simulink library "LinkLib"  (R2023b)
settings: Solver=VariableStepAuto  StartTime=0.0  StopTime=10.0  RelTol=1e-3
undefined symbols (not defined in the file): LpinL, X, Y, Z
libraries: sm_lib x73, $bdroot x2
(part 1 of 3)
settings Model: Creator=abirdas  LastModifiedBy=abirdas

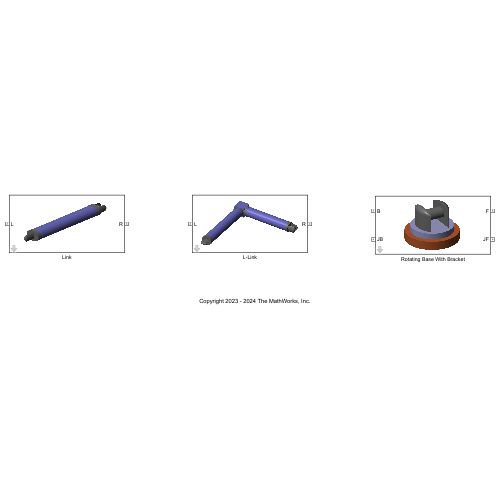
[thumbnail: Simulink's stored preview of the top-level diagram]
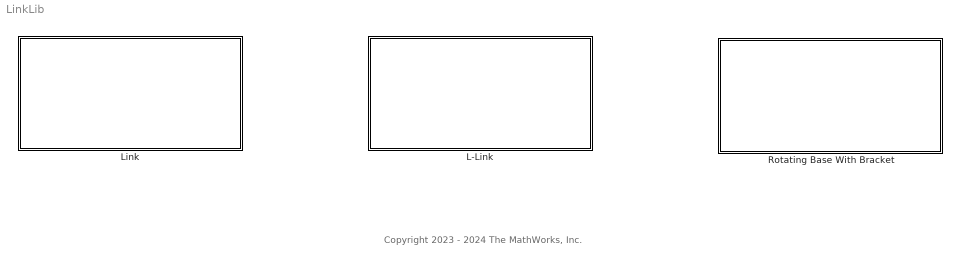
== system LinkLib ==
  note: Copyright 2023 - 2024 The MathWorks, Inc.
  L-Link : Subsystem  mask(Robot Arm L-Link){connConfigLLLink=Single bracket, oriLLLink=+X, connConfigRLLink=Double bracket with pin, oriRLLink=+Z, linkRadius=0.01, member1TotalLength=0.1, member2TotalLength=0.2, inertiaType=Custom, linkMass=0.1, linkCM=[0 0 0], linkMOI=[1 1 1], linkPOI=[0 0 0], linkDensity=7780, linkColor=[0.5 0.5 0.9]}
      mask prompts: connConfigLLLink "Left connector configuration"; oriLLLink "Left bracket orientation"; connConfigRLLink "Right connector configuration"; oriRLLink "Right bracket orientation"; linkRadius "Link radius (m)"; member1TotalLength "Member1 total length (m)"; member2TotalLength "Member 2 total length (m)"; inertiaType "Inertia type"; linkMass "Mass (kg)"; linkCM "Center of mass (m)"; linkMOI "Moments of inertia (kg*m^2)"; linkPOI "Products of inertia (kg*m^2)"; linkDensity "Link density (kg/m^3)"; linkColor "Link color"
      mask help:
      | Consists of two perpendicular members rigidly connected to one another using a rigid middle connector. Each member represents a robot arm link that consists of a middle section, two end plates (left plate and right plate) and two end connectors (left connector and right connector). These components are rigidly connected to one another. The first member or Member 1 is a link with No connector as the right connector. The second member or Member 2 is a link with No connector as the left connector.
      |
      | Attachment points are:
      | L: Left connector
      | R: Right connector
      |
      | Connectors can be of following types:
      | No connector
      | Single bracket
      | Double bracket with pin
      | Rotating pin
      | Pin socket
      |
      | Where
      | Link radius: Radius of the cylinders that constitute the middle section of the links representing Member 1 and Member 2
      | Member1 total length: Distance between the center of left connector of Member 1 and the center of rigid middle connector
      | Member2 total length: Distance between the center of rigid middle connector and the center of right connector of Member 2
      mask init:
      | linkRadius = get_param(gcb,'value@linkRadius');
      | member1TotalLength = get_param(gcb,'value@member1TotalLength');
      | member1Path = [gcb,'/Member 1'];
      | member2TotalLength = get_param(gcb,'value@member2TotalLength');
      | member2Path = [gcb,'/Member 2'];
      | rigidMiddleConnPath = [gcb,'/Rigid Middle Connector'];
      | member1Length = member1TotalLength - 1.05*linkRadius;
      | middleConnL = 2*1.05*linkRadius;
      | set_param(member1Path,'linkRadius',num2str(linkRadius));
      | set_param(member1Path,'linkLength',num2str(member1Length));
      | set_param(rigidMiddleConnPath,'midConnL',num2str(middleConnL));
      | member2Length = member2TotalLength - 1.05*linkRadius;
      | set_param(member2Path,'linkRadius',num2str(linkRadius));
      | set_param(member2Path,'linkLength',num2str(member2Length))
      mask Help: web('LLink.html')
      mask TypeOptions connConfigLLLink: No connector | Single bracket | Double bracket with pin | Rotating pin | Pin socket
      mask Callback connConfigLLLink:
      | maskObj = Simulink.Mask.get(gcb);
      | connConfigLLLink = maskObj.getParameter('connConfigLLLink');
      | oriLLLink = maskObj.getParameter('oriLLLink');
      | member1Path = [gcb,'/Member 1'];
      | if strcmp(connConfigLLLink.Value,'No connector') || ...
      |         strcmp(connConfigLLLink.Value,'Rotating pin') || ...
      |         strcmp(connConfigLLLink.Value,'Pin socket')
      |     oriLLLink.Visible = 'off';
      | else
      |     oriLLLink.Visible = 'on';
      | end
      | set_param(member1Path,'connConfigL',connConfigLLLink.Value);
      | set_param(member1Path,'oriL',oriLLLink.Value);
      | set_param(member1Path,'connConfigR','No connector');
      mask TypeOptions oriLLLink: +X | +Z
      mask TypeOptions connConfigRLLink: No connector | Single bracket | Double bracket with pin | Rotating pin | Pin socket
      mask Callback connConfigRLLink:
      | maskObj = Simulink.Mask.get(gcb);
      | connConfigRLLink = maskObj.getParameter('connConfigRLLink');
      | oriRLLink = maskObj.getParameter('oriRLLink');
      | member2Path = [gcb,'/Member 2'];
      | if strcmp(connConfigRLLink.Value,'No connector') || ...
      |         strcmp(connConfigRLLink.Value,'Rotating pin') || ...
      |         strcmp(connConfigRLLink.Value,'Pin socket')
      |     oriRLLink.Visible = 'off';
      | else
      |     oriRLLink.Visible = 'on';
      | end
      | set_param(member2Path,'connConfigR',connConfigRLLink.Value);
      | if strcmp(oriRLLink.Value,'+Z')
      |     set_param(member2Path,'oriR',oriRLLink.Value);
      | elseif strcmp(oriRLLink.Value,'+Y')
      |     set_param(member2Path,'oriR','+X');
      | end
      | set_param(member2Path,'connConfigL','No connector');
      mask TypeOptions oriRLLink: +Y | +Z
      mask TypeOptions inertiaType: Calculate from geometry | Custom
      mask Callback inertiaType:
      | maskObj = Simulink.Mask.get(gcb);
      | inertiaTypeLLink = maskObj.getParameter('inertiaType');
      | massLLink = maskObj.getParameter('linkMass');
      | centerOfMassLLink = maskObj.getParameter('linkCM');
      | momentsOfInertiaLLink = maskObj.getParameter('linkMOI');
      | productsOfInertiaLLink = maskObj.getParameter('linkPOI');
      | linkDensityLLink = maskObj.getParameter('linkDensity');
      | linkColorLLink = maskObj.getParameter('linkColor');
      | linkRadius = maskObj.getParameter('linkRadius');
      | member1Path = [gcb,'/Member 1'];
      | member2Path = [gcb,'/Member 2'];
      | rigidMiddleConnPath = [gcb,'/Rigid Middle Connector/Brick Solid'];
      | if strcmp(inertiaTypeLLink.Value,'Calculate from geometry')
      |     massLLink.Visible='off';
      |     centerOfMassLLink.Visible='off';
      |     momentsOfInertiaLLink.Visible='off';
      |     productsOfInertiaLLink.Visible='off';
      |     linkDensityLLink.Visible='on';
      |     set_param(rigidMiddleConnPath,'InertiaType','CalculateFromGeometry');
      |     set_param(rigidMiddleConnPath,'BasedOnType','Density');
      | elseif strcmp(inertiaTypeLLink.Value,'Custom')
      |     massLLink.Visible='on';
      |     centerOfMassLLink.Visible='on';
      |     momentsOfInertiaLLink.Visible='on';
      |     productsOfInertiaLLink.Visible='on';
      |     linkDensityLLink.Visible='off';
      |     set_param(rigidMiddleConnPath,'InertiaType','Custom');
      | end
      | 
      | set_param(member1Path,'inertiaType',inertiaTypeLLink.Value);
      | set_param(member1Path,'linkMass',massLLink.Value);
      | set_param(member1Path,'linkCM',centerOfMassLLink.Value);
      | set_param(member1Path,'linkMOI',momentsOfInertiaLLink.Value);
      | set_param(member1Path,'linkPOI',productsOfInertiaLLink.Value);
      | set_param(member1Path,'linkDensity',linkDensityLLink.Value);
      | set_param(member1Path,'linkColor',linkColorLLink.Value);
      | set_param(member2Path,'linkRadius',linkRadius.Value);
      | set_param(member2Path,'inertiaType',inertiaTypeLLink.Value);
      | set_param(member2Path,'linkMass','1e-10');
      | set_param(member2Path,'linkCM','[0 0 0]');
      | set_param(member2Path,'linkMOI','[0 0 0]');
      | set_param(member2Path,'linkPOI','[0 0 0]');
      | set_param(member2Path,'linkDensity',linkDensityLLink.Value);
      | set_param(member2Path,'linkColor',linkColorLLink.Value);
      mask DialogControl Container1 Prompt: Connector configuration
      mask DialogControl Container2 Prompt: Geometry
      mask DialogControl Container3 Prompt: Inertia
      mask DialogControl Container4 Prompt: Graphic
      mask Display:
      | image('LLinkIcon.png');
      | port_label('lconn',1,'L');
      | port_label('rconn',1,'R');
  Link : Subsystem  mask(Robot Arm Link){connConfigL=Single bracket, oriL=+X, connConfigR=Double bracket with pin, oriR=+X, linkRadius=0.01, linkLength=0.1, inertiaType=Custom, linkMass=3, linkCM=[0 0 0], linkMOI=[1 1 1], linkPOI=[0 0 0], linkDensity=7780, linkColor=[0.5, 0.5, 0.88]}
      mask prompts: connConfigL "Left connector configuration"; oriL "Left bracket orientation"; connConfigR "Right connector configuration"; oriR "Right bracket orientation"; linkRadius "Link radius (m)"; linkLength "Link length (m)"; inertiaType "Inertia type"; linkMass "Mass (kg)"; linkCM "Center of mass (m)"; linkMOI "Moments of inertia (kg*m^2)"; linkPOI "Products of inertia (kg*m^2)"; linkDensity "Link density (kg//m^3)"; linkColor "Link color"
      mask help:
      | Consists of a cylindrical middle section, two end plates (left plate and right plate) and two end connectors (left connector and right connector). These components are rigidly connected to one another.
      |
      | Attachment points are:
      | L: Left connector
      | R: Right connector
      |
      | Connectors can be of following types:
      | No connector
      | Single bracket
      | Double bracket with pin
      | Rotating pin
      | Pin socket
      |
      | Where
      | Link radius: Radius of the cylinder that constitutes the middle section of the link
      | Link length: Distance between the center of left connector and the center of right connector of the link
      mask init:
      | maskObj = Simulink.Mask.get(gcb);
      | connConfigL = maskObj.getParameter('connConfigL');
      | connConfigR = maskObj.getParameter('connConfigR');
      | linkRadius = get_param(gcb,'value@linkRadius');
      | linkLength = get_param(gcb,'value@linkLength');
      | bracketLength = (linkRadius/2)*1.5;
      | pinLength = linkRadius/2;
      | midSecPath = [gcb,'/Middle Section'];
      | leftPlatePath = [gcb,'/Left Plate'];
      | rightPlatePath = [gcb,'/Right Plate'];
      | if strcmp(connConfigL.Value, 'Single bracket') || strcmp(connConfigL.Value,'Double bracket with pin')
      |     if strcmp(connConfigR.Value, 'Single bracket') || strcmp(connConfigR.Value,'Double bracket with pin')
      |         midSecLength = (linkLength - 2*bracketLength)/(1 + 2*0.05);
      |     elseif strcmp(connConfigR.Value, 'Rotating pin') || strcmp(connConfigR.Value,'Pin socket')
      |         midSecLength= (linkLength - bracketLength - 0.5*pinLength)/(1 + 2*0.05);
      |     elseif strcmp(connConfigR.Value, 'No connector')
      |         midSecLength= (linkLength - bracketLength)/(1 + 2*0.05);
      |     end
      | elseif strcmp(connConfigL.Value, 'Rotating pin') || strcmp(connConfigL.Value,'Pin socket')
      |     if strcmp(connConfigR.Value, 'Single bracket') || strcmp(connConfigR.Value,'Double bracket with pin')
      |         midSecLength= (linkLength - bracketLength - 0.5*pinLength)/(1 + 2*0.05);
      |     elseif strcmp(connConfigR.Value, 'Rotating pin') || strcmp(connConfigR.Value,'Pin socket')
      |         midSecLength = (linkLength - 2*0.5*pinLength)/(1 + 2*0.05);
      |     elseif strcmp(connConfigR.Value, 'No connector')
      |         midSecLength = (linkLength - 0.5*pinLength)/(1 + 2*0.05);
      |     end
      | elseif strcmp(connConfigL.Value, 'No connector')
      |     if strcmp(connConfigR.Value, 'Single bracket') || strcmp(connConfigR.Value,'Double bracket with pin')
      |         midSecLength= (linkLength - bracketLength)/(1 + 2*0.05);
      |     elseif strcmp(connConfigR.Value, 'Rotating pin') || strcmp(connConfigR.Value,'Pin socket')
      |         midSecLength = (linkLength - 0.5*pinLength)/(1 + 2*0.05);
      |     elseif strcmp(connConfigR.Value, 'No connector')
      |         midSecLength = (linkLength)/(1 + 2*0.05);
      |     end
      | end
      | set_param(midSecPath, 'midSecLength', num2str(midSecLength));
      | set_param(leftPlatePath, 'plateThickness', num2str(0.05*midSecLength));
      | set_param(rightPlatePath, 'plateThickness', num2str(0.05*midSecLength));
      mask Help: web('Link.html')
      mask TypeOptions connConfigL: No connector | Single bracket | Double bracket with pin | Rotating pin | Pin socket
      mask Callback connConfigL:
      | maskObj = Simulink.Mask.get(gcb);
      | connConfigL = maskObj.getParameter('connConfigL');
      | oriL = maskObj.getParameter('oriL');
      | blockPath = [gcb,'/Left Connector'];
      | transformBracketPathL = [gcb,'/Left Connector/Bracket/Bracket/Transform Bracket L'];
      | transformBracketPathR = [gcb,'/Left Connector/Bracket/Bracket/Transform Bracket R'];
      | pinBracketPath = [gcb,'/Left Connector/Bracket/Pin B'];
      | if strcmp(connConfigL.Value,'No connector')
      |     oriL.Visible='off';
      |     set_param(blockPath, 'LabelModeActiveChoice', 'NoConnectorL');
      | elseif strcmp(connConfigL.Value,'Single bracket')
      |     oriL.Visible='on';
      |     set_param(blockPath, 'LabelModeActiveChoice', 'BracketL');
      |     set_param(pinBracketPath,'commented','through');
      |     set_param(transformBracketPathL,'TranslationStandardOffset','0');
      |     set_param(transformBracketPathR,'TranslationStandardOffset','0');
      | elseif strcmp(connConfigL.Value,'Double bracket with pin')
      |     oriL.Visible='on';
      |     set_param(blockPath, 'LabelModeActiveChoice', 'BracketL');
      |     set_param(pinBracketPath,'commented','off');
      |     set_param(transformBracketPathL,'TranslationStandardOffset','wBracket/2');
      |     set_param(transformBracketPathR,'TranslationStandardOffset','wBracket/2');
      | elseif strcmp(connConfigL.Value,'Rotating pin')
      |     oriL.Visible='off';
      |     set_param(blockPath, 'LabelModeActiveChoice', 'RotatingPinL');
      | elseif strcmp(connConfigL.Value,'Pin socket')
      |     oriL.Visible='off';
      |     set_param(blockPath, 'LabelModeActiveChoice', 'PinSocketL');
      | end
      mask TypeOptions oriL: +X | +Z
      mask TypeOptions connConfigR: No connector | Single bracket | Double bracket with pin | Rotating pin | Pin socket
      mask Callback connConfigR:
      | maskObj = Simulink.Mask.get(gcb);
      | connConfigR = maskObj.getParameter('connConfigR');
      | oriR = maskObj.getParameter('oriR');
      | blockPath = [gcb,'/Right Connector'];
      | transformBracketPathL = [gcb,'/Right Connector/Bracket/Bracket/Transform Bracket L'];
      | transformBracketPathR = [gcb,'/Right Connector/Bracket/Bracket/Transform Bracket R'];
      | 
      | pinBracketPath = [gcb,'/Right Connector/Bracket/Pin B'];
      | if strcmp(connConfigR.Value,'No connector')
      |     oriR.Visible='off';
      |     set_param(blockPath, 'LabelModeActiveChoice', 'NoConnectorR');
      | elseif strcmp(connConfigR.Value,'Single bracket')
      |     oriR.Visible='on';
      |     set_param(blockPath, 'LabelModeActiveChoice', 'BracketR');
      |     set_param(pinBracketPath,'commented','through');
      |     set_param(transformBracketPathL,'TranslationStandardOffset','0');
      |     set_param(transformBracketPathR,'TranslationStandardOffset','0');
      | elseif strcmp(connConfigR.Value,'Double bracket with pin')
      |     oriR.Visible='on';
      |     set_param(blockPath, 'LabelModeActiveChoice', 'BracketR');
      |     set_param(pinBracketPath,'commented','off');
      |     set_param(transformBracketPathL,'TranslationStandardOffset','wBracket/2');
      |     set_param(transformBracketPathR,'TranslationStandardOffset','wBracket/2');
      | elseif strcmp(connConfigR.Value,'Rotating pin')
      |     oriR.Visible='off';
      |     set_param(blockPath, 'LabelModeActiveChoice', 'RotatingPinR');
      | elseif strcmp(connConfigR.Value,'Pin socket')
      |     oriR.Visible='off';
      |     set_param(blockPath, 'LabelModeActiveChoice', 'PinSocketR');
      | end
      mask TypeOptions oriR: +X | +Z
      mask Callback oriR:
      | maskObj = Simulink.Mask.get(gcb);
      | blockPath = gcb;
      | connConfigL = maskObj.getParameter('connConfigL');
      | connConfigR = maskObj.getParameter('connConfigR');
      | oriR = maskObj.getParameter('oriR');
      | oriL = maskObj.getParameter('oriL');
      | 
      | transformLXPath = [blockPath,'/Transform LX'];
      | transformLZPath = [blockPath,'/Transform LZ'];
      | transformRB1Path = [blockPath,'/Transform RB1'];
      | transformRB2Path = [blockPath,'/Transform RB2'];
      | transformRFPath = [blockPath,'/Transform RF'];
      | 
      | if strcmp(connConfigL.Value,'Single bracket') || ...
      |         strcmp(connConfigL.Value,'Double bracket with pin')
      | if strcmp(connConfigR.Value,'Single bracket') || ...
      |         strcmp(connConfigR.Value,'Double bracket with pin')
      | if strcmp(oriL.Value,'+X') && strcmp(oriR.Value,'+X')
      |     set_param(transformLXPath,'commented','off');
      |     set_param(transformLZPath,'commented','through');
      |     set_param(transformRB1Path,'commented','off');
      |     set_param(transformRB2Path,'commented','through');
      |     set_param(transformRFPath,'commented','off');
      | elseif strcmp(oriL.Value,'+X') && strcmp(oriR.Value,'+Z')
      |     set_param(transformLXPath,'commented','off');
      |     set_param(transformLZPath,'commented','through');
      |     set_param(transformRB1Path,'commented','through');
      |     set_param(transformRB2Path,'commented','off');
      |     set_param(transformRFPath,'commented','through');
      | elseif strcmp(oriL.Value,'+Z') && strcmp(oriR.Value,'+X')
      |     set_param(transformLXPath,'commented','through');
      |     set_param(transformLZPath,'commented','off');
      |     set_param(transformRB1Path,'commented','through');
      |     set_param(transformRB2Path,'commented','off');
      |     set_param(transformRFPath,'commented','off');
      | elseif strcmp(oriL.Value,'+Z') && strcmp(oriR.Value,'+Z')
      |     set_param(transformLXPath,'commented','through');
      |     set_param(transformLZPath,'commented','off');
      |     set_param(transformRB1Path,'commented','off');
      |     set_param(transformRB2Path,'commented','through');
      |     set_param(transformRFPath,'commented','through');
      | end
      | elseif strcmp(connConfigR.Value,'No connector') || ...
      |         strcmp(connConfigR.Value,'Rotating pin') || ...
      |         strcmp(connConfigR.Value,'Pin socket')
      |     if strcmp(oriL.Value,'+X')
      |     set_param(transformLXPath,'commented','off');
      |     set_param(transformLZPath,'commented','through');
      |     set_param(transformRB1Path,'commented','off');
      |     set_param(transformRB2Path,'commented','through');
      |     set_param(transformRFPath,'commented','off');
      |     elseif strcmp(oriL.Value,'+Z')
      |     set_param(transformLXPath,'commented','through');
      |     set_param(transformLZPath,'commented','off');
      |     set_param(transformRB1Path,'commented','through');
      |     set_param(transformRB2Path,'commented','off');
      |     set_param(transformRFPath,'commented','off');
      |     end
      | end
      | elseif strcmp(connConfigL.Value,'No connector') || ...
      |         strcmp(connConfigL.Value,'Rotating pin') || ...
      |         strcmp(connConfigL.Value,'Pin socket')
      |     if strcmp(connConfigR.Value,'Single bracket') || ...
      |         strcmp(connConfigR.Value,'Double bracket with pin')
      |     if strcmp(oriR.Value,'+X')
      |     set_param(transformLXPath,'commented','off');
      |     set_param(transformLZPath,'commented','through');
      |     set_param(transformRB1Path,'commented','off');
      |     set_param(transformRB2Path,'commented','through');
      |     set_param(transformRFPath,'commented','off');
      |     elseif strcmp(oriR.Value,'+Z')
      |     set_param(transformLXPath,'commented','off');
      |     set_param(transformLZPath,'commented','through');
      |     set_param(transformRB1Path,'commented','through');
      |     set_param(transformRB2Path,'commented','off');
      |     set_param(transformRFPath,'commented','through');
      |     end
      | elseif strcmp(connConfigR.Value,'No connector') || ...
      |         strcmp(connConfigR.Value,'Rotating pin') || ...
      |         strcmp(connConfigR.Value,'Pin socket')
      |     set_param(transformLXPath,'commented','off');
      |     set_param(transformLZPath,'commented','through');
      |     set_param(transformRB1Path,'commented','off');
      |     set_param(transformRB2Path,'commented','through');
      |     set_param(transformRFPath,'commented','off');
      |     end
      | end
      mask TypeOptions inertiaType: Calculate from Geometry | Custom
      mask Callback inertiaType:
      | maskObj = Simulink.Mask.get(gcb);
      | inertiaType = maskObj.getParameter('inertiaType');
      | mass = maskObj.getParameter('linkMass');
      | centerOfMass = maskObj.getParameter('linkCM');
      | momentsOfInertia = maskObj.getParameter('linkMOI');
      | productsOfInertia = maskObj.getParameter('linkPOI');
      | linkDensity = maskObj.getParameter('linkDensity');
      | leftBracketLSolid1Path = [gcb,'/Left Connector/Bracket/Bracket/BracketL/Extruded Solid'];
      | leftBracketLSolid2Path = [gcb,'/Left Connector/Bracket/Bracket/BracketL/Revolved Solid'];
      | leftBracketRSolid1Path = [gcb,'/Left Connector/Bracket/Bracket/BracketR/Extruded Solid'];
      | leftBracketRSolid2Path = [gcb,'/Left Connector/Bracket/Bracket/BracketR/Revolved Solid'];
      | leftBracketPinPath = [gcb,'/Left Connector/Bracket/Pin B/Cylindrical Solid'];
      | leftRotatingPinPath = [gcb,'/Left Connector/Rotating Pin/Cylindrical Solid'];
      | leftPinSocketPath = [gcb,'/Left Connector/Pin Socket/Bar'];
      | leftPlatePath = [gcb,'/Left Plate/Cylindrical Solid'];
      | midSecPath = [gcb,'/Middle Section/Cylindrical Solid'];
      | rightPlatePath = [gcb,'/Right Plate/Cylindrical Solid'];
      | rightBracketLSolid1Path = [gcb,'/Right Connector/Bracket/Bracket/BracketL/Extruded Solid'];
      | rightBracketLSolid2Path = [gcb,'/Right Connector/Bracket/Bracket/BracketL/Revolved Solid'];
      | rightBracketRSolid1Path = [gcb,'/Right Connector/Bracket/Bracket/BracketR/Extruded Solid'];
      | rightBracketRSolid2Path = [gcb,'/Right Connector/Bracket/Bracket/BracketR/Revolved Solid'];
      | rightBracketPinPath = [gcb,'/Right Connector/Bracket/Pin B/Cylindrical Solid'];
      | rightRotatingPinPath = [gcb,'/Right Connector/Rotating Pin/Cylindrical Solid'];
      | rightPinSocketPath = [gcb,'/Right Connector/Pin Socket/Bar'];
      | 
      | if strcmp(inertiaType.Value,'Calculate from Geometry')
      |     mass.Visible='off';
      |     centerOfMass.Visible='off';
      |     momentsOfInertia.Visible='off';
      |     productsOfInertia.Visible='off';
      |     linkDensity.Visible='on';
      |     set_param(leftBracketLSolid1Path,'InertiaType','CalculateFromGeometry');
      |     set_param(leftBracketLSolid1Path,'BasedOnType','Density');
      |     set_param(leftBracketLSolid2Path,'InertiaType','CalculateFromGeometry');
      |     set_param(leftBracketLSolid2Path,'BasedOnType','Density');
      |     set_param(leftBracketRSolid1Path,'InertiaType','CalculateFromGeometry');
      |     set_param(leftBracketRSolid1Path,'BasedOnType','Density');
      |     set_param(leftBracketRSolid2Path,'InertiaType','CalculateFromGeometry');
      |     set_param(leftBracketRSolid2Path,'BasedOnType','Density');
      |     set_param(leftBracketPinPath,'InertiaType','CalculateFromGeometry');
      |     set_param(leftBracketPinPath,'BasedOnType','Density');
      |     set_param(leftRotatingPinPath,'InertiaType','CalculateFromGeometry');
      |     set_param(leftRotatingPinPath,'BasedOnType','Density');
      |     set_param(leftPinSocketPath,'InertiaType','CalculateFromGeometry');
      |     set_param(leftPinSocketPath,'BasedOnType','Density');
      |     set_param(leftPlatePath,'InertiaType','CalculateFromGeometry');
      |     set_param(leftPlatePath,'BasedOnType','Density');
      |     set_param(midSecPath,'InertiaType','CalculateFromGeometry');
      |     set_param(midSecPath,'BasedOnType','Density');
      |     set_param(rightPlatePath,'InertiaType','CalculateFromGeometry');
      |     set_param(rightPlatePath,'BasedOnType','Density');
      |     set_param(rightBracketLSolid1Path,'InertiaType','CalculateFromGeometry');
      |     set_param(rightBracketLSolid1Path,'BasedOnType','Density');
      |     set_param(rightBracketLSolid2Path,'InertiaType','CalculateFromGeometry');
      |     set_param(rightBracketLSolid2Path,'BasedOnType','Density');
      |     set_param(rightBracketRSolid1Path,'InertiaType','CalculateFromGeometry');
      |     set_param(rightBracketRSolid1Path,'BasedOnType','Density');
      |     set_param(rightBracketRSolid2Path,'InertiaType','CalculateFromGeometry');
      |     set_param(rightBracketRSolid2Path,'BasedOnType','Density');
      |     set_param(rightBracketPinPath,'InertiaType','CalculateFromGeometry');
      |     set_param(rightBracketPinPath,'BasedOnType','Density');
      |     set_param(rightRotatingPinPath,'InertiaType','CalculateFromGeometry');
      |     set_param(rightRotatingPinPath,'BasedOnType','Density');
      |     set_param(rightPinSocketPath,'InertiaType','CalculateFromGeometry');
      |     set_param(rightPinSocketPath,'BasedOnType','Density');
      | elseif strcmp(inertiaType.Value,'Custom')
      |     mass.Visible='on';
      |     centerOfMass.Visible='on';
      |     momentsOfInertia.Visible='on';
      |     productsOfInertia.Visible='on';
      |     linkDensity.Visible='off';
      |     set_param(leftBracketLSolid1Path,'InertiaType','Custom');
      |     set_param(leftBracketLSolid2Path,'InertiaType','Custom');
      |     set_param(leftBracketRSolid1Path,'InertiaType','Custom');
      |     set_param(leftBracketRSolid2Path,'InertiaType','Custom');
      |     set_param(leftBracketPinPath,'InertiaType','Custom');
      |     set_param(leftRotatingPinPath,'InertiaType','Custom');
      |     set_param(leftPinSocketPath,'InertiaType','Custom');
      |     set_param(leftPlatePath,'InertiaType','Custom');
      |     set_param(midSecPath,'InertiaType','Custom');
      |     set_param(rightPlatePath,'InertiaType','Custom');
      |     set_param(rightBracketLSolid1Path,'InertiaType','Custom');
      |     set_param(rightBracketLSolid2Path,'InertiaType','Custom');
      |     set_param(rightBracketRSolid1Path,'InertiaType','Custom');
      |     set_param(rightBracketRSolid2Path,'InertiaType','Custom');
      |     set_param(rightBracketPinPath,'InertiaType','Custom');
      |     set_param(rightRotatingPinPath,'InertiaType','Custom');
      |     set_param(rightPinSocketPath,'InertiaType','Custom');
      | end
      mask DialogControl Container1 Prompt: Connector configuration
      mask DialogControl Container2 Prompt: Geometry
      mask DialogControl Container3 Prompt: Inertia
      mask DialogControl Container4 Prompt: Graphic
      mask Display:
      | image('LinkIcon.PNG');
      | port_label('lconn',1,'L');
      | port_label('rconn',1,'R');
  Rotating Base With Bracket : Subsystem  mask(Rotating Base With Bracket){connConfig=Single bracket, baseRadius=0.01, baseTotalLength=0.05, baseInertiaType=Custom, baseDensity=7780, baseMass=5, baseCM=[0 0 0], baseMOI=[1 1 1], basePOI=[0 0 0], rotorInertiaType=Custom, rotorDensity=7780, rotorMass=3, rotorCM=[0 0 0], rotorMOI=[1 1 1], rotorPOI=[0 0 0], baseColor=[0.8 0.4 0.2], rotorColor=[0.7 0.7 0.9]}
      mask prompts: connConfig "Bracket configuration"; baseRadius "Fixed base radius (m)"; baseTotalLength "Base total length (m)"; baseInertiaType "Inertia type"; baseDensity "Density (kg/m^3)"; baseMass "Mass (kg)"; baseCM "Center of mass (m)"; baseMOI "Moments of inertia (kg*m^2)"; basePOI "Products of inertia (kg*m^2)"; rotorInertiaType "Inertia type"; rotorDensity "Density (kg/m^3)"; rotorMass "Mass (kg)"; rotorCM "Center of mass (m)"; rotorMOI "Moments of inertia (kg*m^2)"; rotorPOI "Products of inertia (kg*m^2)"; baseColor "Fixed base color"; rotorColor "Rotor color"
      mask help:
      | Consists of a fixed base, a rotor and a bracket mounted on the rotor. The rotor must be connected to the fixed base using a Revolute Joint. The bracket is connected rigidly to the rotor.
      |
      | Attachment points are:
      | B: The bottom of the fixed base
      | F: The center point of the hole or between the two holes of the bracket.
      | JB: The top of the fixed base, which is attached to the bottom of the rotor.
      | JF: The bottom of the rotor, which is attached to the top of the fixed base.
      | All attachments are configured for Revolute joints.
      |
      | Bracket can be of following types:
      | Single bracket
      | Double bracket with pin
      |
      | Where
      | Fixed base radius: Radius of the cylinder that constitutes the fixed base
      | Base total length: Distance between the bottom surface of the fixed base and the center of hole (for Single bracket) or center of pin (for Double bracket with pin) of the bracket, measured in the direction perpendicular to the bottom surface of the fixed base
      mask init:
      | baseTotalLength = get_param(gcb,'value@baseTotalLength');
      | baseRadius = get_param(gcb,'value@baseRadius');
      | rotorRadius = 0.8*baseRadius;
      | bracketLength = (rotorRadius/2)*1.5;
      | baseLength = (baseTotalLength - bracketLength)/1.7;
      | rotorLength = 0.7*baseLength;
      | basePath = [gcb,'/Fixed Base'];
      | rotorPath = [gcb,'/Rotor'];
      | set_param(basePath, 'CylinderLength', num2str(baseLength));
      | set_param(rotorPath, 'CylinderLength', num2str(rotorLength));
      mask Help: web('RotatingBaseWithBracket.html')
      mask TypeOptions connConfig: Double bracket with pin | Single bracket
      mask Callback connConfig:
      | maskObj = Simulink.Mask.get(gcb);
      | connConfig = maskObj.getParameter('connConfig');
      | pinBracketPath = [gcb,'/Bracket/Pin B'];
      | transformBracketPathL = [gcb,'/Bracket/Bracket/Transform Bracket L'];
      | transformBracketPathR = [gcb,'/Bracket/Bracket/Transform Bracket R'];
      | switch connConfig.Value
      |     case 'Single bracket'
      |         set_param(pinBracketPath,'commented','through');
      |         set_param(transformBracketPathL,'TranslationStandardOffset','0');
      |         set_param(transformBracketPathR,'TranslationStandardOffset','0');
      |     case 'Double bracket with pin'
      |         set_param(pinBracketPath,'commented','off');
      |         set_param(transformBracketPathL,'TranslationStandardOffset','wBracket/2');
      |         set_param(transformBracketPathR,'TranslationStandardOffset','wBracket/2');
      | end
      mask TypeOptions baseInertiaType: Calculate from geometry | Custom
      mask Callback baseInertiaType:
      | maskObj = Simulink.Mask.get(gcb);
      | baseInertiaType = maskObj.getParameter('baseInertiaType');
      | baseDensity= maskObj.getParameter('baseDensity');
      | baseMass= maskObj.getParameter('baseMass');
      | baseCM= maskObj.getParameter('baseCM');
      | baseMOI= maskObj.getParameter('baseMOI');
      | basePOI= maskObj.getParameter('basePOI');
      | basePath = [gcb,'/Fixed Base'];
      | switch baseInertiaType.Value
      |     case 'Calculate from geometry'
      |         baseDensity.Visible='on';
      | 		baseMass.Visible='off';
      | 		baseCM.Visible='off';
      | 		baseMOI.Visible='off';
      | 		basePOI.Visible='off';
      |         set_param(basePath,'InertiaType','CalculateFromGeometry');
      |         set_param(basePath, 'BasedOnType', 'Density');
      |     case 'Custom'
      |         baseDensity.Visible='off';
      | 		baseMass.Visible='on';
      | 		baseCM.Visible='on';
      | 		baseMOI.Visible='on';
      | 		basePOI.Visible='on';
      |         set_param(basePath,'InertiaType','Custom');
      | end
      mask TypeOptions rotorInertiaType: Calculate from geometry | Custom
      mask Callback rotorInertiaType:
      | maskObj = Simulink.Mask.get(gcb);
      | rotorInertiaType = maskObj.getParameter('rotorInertiaType');
      | rotorDensity= maskObj.getParameter('rotorDensity');
      | rotorMass= maskObj.getParameter('rotorMass');
      | rotorCM= maskObj.getParameter('rotorCM');
      | rotorMOI= maskObj.getParameter('rotorMOI');
      | rotorPOI= maskObj.getParameter('rotorPOI');
      | rotorPath = [gcb,'/Rotor'];
      | bracketLSolid1Path = [gcb,'/Bracket/Bracket/BracketL/Extruded Solid'];
      | bracketLSolid2Path = [gcb,'/Bracket/Bracket/BracketL/Revolved Solid'];
      | bracketRSolid1Path = [gcb,'/Bracket/Bracket/BracketR/Extruded Solid'];
      | bracketRSolid2Path = [gcb,'/Bracket/Bracket/BracketR/Revolved Solid'];
      | bracketPinPath = [gcb,'/Bracket/Pin B/Cylindrical Solid'];
      | 
      | switch rotorInertiaType.Value
      |     case 'Calculate from geometry'
      |         rotorDensity.Visible='on';
      | 		rotorMass.Visible='off';
      | 		rotorCM.Visible='off';
      | 		rotorMOI.Visible='off';
      | 		rotorPOI.Visible='off';
      |         set_param(rotorPath,'InertiaType','CalculateFromGeometry');
      |         set_param(rotorPath, 'BasedOnType', 'Density');
      |         set_param(bracketLSolid1Path,'InertiaType','CalculateFromGeometry');
      |         set_param(bracketLSolid1Path, 'BasedOnType', 'Density');
      |         set_param(bracketLSolid2Path,'InertiaType','CalculateFromGeometry');
      |         set_param(bracketLSolid2Path, 'BasedOnType', 'Density');
      |         set_param(bracketRSolid1Path,'InertiaType','CalculateFromGeometry');
      |         set_param(bracketRSolid1Path, 'BasedOnType', 'Density');
      |         set_param(bracketRSolid2Path,'InertiaType','CalculateFromGeometry');
      |         set_param(bracketRSolid2Path, 'BasedOnType', 'Density');
      |         set_param(bracketPinPath,'InertiaType','CalculateFromGeometry');
      |         set_param(bracketPinPath, 'BasedOnType', 'Density');
      |     case 'Custom'
      |         rotorDensity.Visible='off';
      | 		rotorMass.Visible='on';
      | 		rotorCM.Visible='on';
      | 		rotorMOI.Visible='on';
      | 		rotorPOI.Visible='on';
      |         set_param(rotorPath,'InertiaType','Custom');
      |         set_param(bracketLSolid1Path,'InertiaType','Custom');
      |         set_param(bracketLSolid2Path,'InertiaType','Custom');
      |         set_param(bracketRSolid1Path,'InertiaType','Custom');
      |         set_param(bracketRSolid2Path,'InertiaType','Custom');
      |         set_param(bracketPinPath,'InertiaType','Custom');
      | end
      mask DialogControl Container1 Prompt: Geometry
      mask DialogControl Container2 Prompt: Inertia
      mask DialogControl BaseCylinder Prompt: Fixed Base
      mask DialogControl Rotor Prompt: Rotor
      mask DialogControl Container3 Prompt: Graphic
      mask Display:
      | image('RotatingBaseWithBracketIcon.PNG');
      | port_label('lconn',1,'B');
      | port_label('rconn',1,'F');
      | port_label('lconn',2,'JB');
      | port_label('rconn',2,'JF');

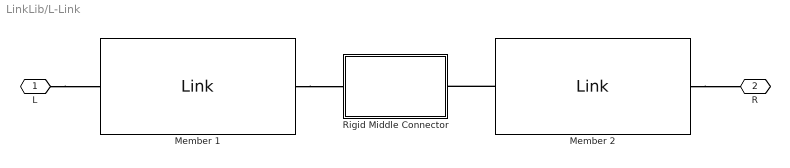
== system LinkLib/L-Link ==
  Member 1 : $bdroot/Link  connConfigL=Single bracket  oriL=+X  connConfigR=No connector  oriR=+X  linkRadius=0.01  linkLength=0.0895  inertiaType=Custom  linkMass=0.1  linkCM=[0 0 0]  linkMOI=[1 1 1]  linkPOI=[0 0 0]  linkDensity=7780  linkColor=[0.5 0.5 0.9]
  Member 2 : $bdroot/Link  connConfigL=No connector  oriL=+X  connConfigR=Double bracket with pin  oriR=+Z  linkRadius=0.01  linkLength=0.1895  inertiaType=Custom  linkMass=1e-10  linkCM=[0 0 0]  linkMOI=[0 0 0]  linkPOI=[0 0 0]  linkDensity=7780  linkColor=[0.5 0.5 0.9]
  Rigid Middle Connector : Subsystem  mask{midConnL=0.021, midConnColor=linkColor}
      mask prompts: midConnL "Middle connector length (m)"; midConnColor "Middle connector color"
      mask Display:
      | image('LLinkRigidMidConnectorIcon.png');
      | port_label('lconn',1,'B');
      | port_label('rconn',1,'F');
  L : PMIOPort  Side=Left
  R : PMIOPort  Port=2  Side=Right
  connections:
  Member 2/RConn1 -- R/RConn1
  Member 1/RConn1 -- Rigid Middle Connector/LConn1
  Member 2/LConn1 -- Rigid Middle Connector/RConn1
  L/RConn1 -- Member 1/LConn1

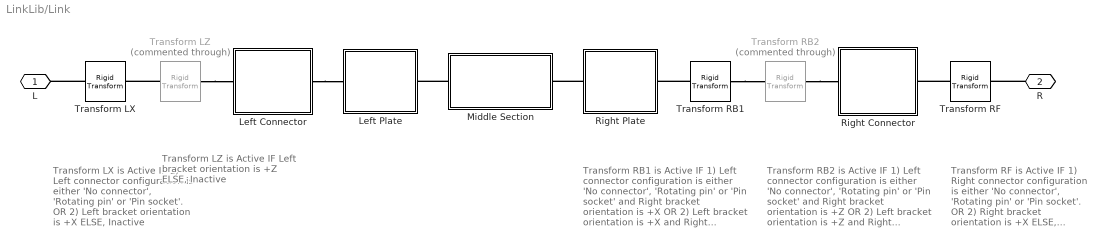
== system LinkLib/Link ==
  note: Transform LX is Active IF
      | 1) Left connector configuration is either 'No connector', 'Rotating pin' or 'Pin socket'.
      | OR
      | 2) Left bracket orientation is +X
      | ELSE,
      | Inactive
  note: Transform LZ is Active IF
      | Left bracket orientation is +Z
      | ELSE,
      | Inactive
  note: Transform RB1 is Active IF
      | 1) Left connector configuration is either 'No connector', 'Rotating pin' or 'Pin socket' and Right bracket orientation is +X
      | OR
      | 2) Left bracket orientation is +X and Right connector configuration is either 'No connector', 'Rotating pin' or 'Pin socket'.
      | OR
      | 3) Left bracket orientation is same as right bracket orientation
      | OR
      | 4) Left connector configuration is either 'No connector', 'Rotating pin' or 'Pin socket' and Right connector configuration is either 'No connector', 'Rotating pin' or 'Pin socket'.
      | ELSE,
      | Inactive
  note: Transform RB2 is Active IF
      | 1) Left connector configuration is either 'No connector', 'Rotating pin' or 'Pin socket' and Right bracket orientation is +Z
      | OR
      | 2) Left bracket orientation is +Z and Right connector configuration is either 'No connector', 'Rotating pin' or 'Pin socket'.
      | OR
      | 3) Left bracket orientation is different than right bracket orientation
      | ELSE,
      | Inactive
  note: Transform RF is Active IF
      | 1) Right connector configuration is either 'No connector', 'Rotating pin' or 'Pin socket'.
      | OR
      | 2) Right bracket orientation is +X
      | ELSE,
      | Inactive
  Left Connector : Subsystem  Variant=on  VariantControlMode=label  LabelModeActiveChoice=BracketL
  Left Plate : Subsystem  mask{plateThickness=0.0038636, plateRadius=1.05*linkRadius, plateColor=[0.5, 0.5, 0.5]}
      mask prompts: plateThickness "Plate thickness (m)"; plateRadius "Plate radius (m)"; plateColor "Plate color"
      mask Display:
      | image('LinkEndPlateIcon.png');
      | port_label('lconn',1,'B');
      | port_label('rconn',1,'F');
  Middle Section : Subsystem  VariantControl=CylindricalSolid  mask{midSecLength=0.077273, midSecRadius=linkRadius, midSecMass=linkMass, midSecCM=linkCM, midSecMOI=linkMOI, midSecPOI=linkPOI, midSecDensity=linkDensity, midSecColor=linkColor}
      mask prompts: midSecLength "Middle section length"; midSecRadius "Middle section radius"; midSecMass "Mass"; midSecCM "Center of mass"; midSecMOI "Moments of inertia"; midSecPOI "Products of inertia"; midSecDensity "Density"; midSecColor "Color"
      mask Display:
      | image('LinkMidSectionIcon.png');
      | port_label('lconn',1,'B');
      | port_label('rconn',1,'F');
  Right Connector : Subsystem  Variant=on  VariantControlMode=label  VariantControl=Choice  LabelModeActiveChoice=BracketR
  Right Plate : Subsystem  mask{plateThickness=0.0038636, plateRadius=1.05*linkRadius, plateColor=[0.5, 0.5, 0.5]}
      mask prompts: plateThickness "Plate thickness (m)"; plateRadius "Plate radius (m)"; plateColor "Plate color"
      mask Display:
      | image('LinkEndPlateIcon.png');
      | port_label('lconn',1,'B');
      | port_label('rconn',1,'F');
  Transform LX : sm_lib/Frames and Transforms/Rigid Transform  TranslationMethod=None  TranslationStandardOffset=0  TranslationStandardOffsetUnits=m  TranslationStandardAxis=+Z  TranslationCartesianOffset=[0 0 0]  TranslationCartesianOffsetUnits=m  TranslationROffset=0  TranslationROffsetUnits=m  TranslationZOffset=0  TranslationZOffsetUnits=m  TranslationThetaOffset=0  TranslationThetaOffsetUnits=deg  RotationMethod=RotationSequence  RotationAngleUnits=deg  RotationStandardAxis=+Z  RotationAngle=180  RotationArbitraryAxis=[0 0 1]  FollAlignAxisA=+X  BaseAlignAxisA=+Y  FollAlignAxisB=+Y  BaseAlignAxisB=+Z  RotationSequenceAxes=BaseAxes  RotationSequence=XYZ  RotationSequenceAngles=[0 90 180]  RotationSequenceAnglesUnits=deg  RotationMatrix=[1 0 0; 0 1 0; 0 0 1]  Quaternion=[1 0 0 0]
  Transform LZ : sm_lib/Frames and Transforms/Rigid Transform  Commented=through  TranslationMethod=None  TranslationStandardOffset=0  TranslationStandardOffsetUnits=m  TranslationStandardAxis=+Z  TranslationCartesianOffset=[0 0 0]  TranslationCartesianOffsetUnits=m  TranslationROffset=0  TranslationROffsetUnits=m  TranslationZOffset=0  TranslationZOffsetUnits=m  TranslationThetaOffset=0  TranslationThetaOffsetUnits=deg  RotationMethod=RotationSequence  RotationAngleUnits=deg  RotationStandardAxis=+Z  RotationAngle=180  RotationArbitraryAxis=[0 0 1]  FollAlignAxisA=+X  BaseAlignAxisA=+Y  FollAlignAxisB=+Y  BaseAlignAxisB=+Z  RotationSequenceAxes=BaseAxes  RotationSequence=XYZ  RotationSequenceAngles=[0 0 180]  RotationSequenceAnglesUnits=deg  RotationMatrix=[1 0 0; 0 1 0; 0 0 1]  Quaternion=[1 0 0 0]
  Transform RB1 : sm_lib/Frames and Transforms/Rigid Transform  TranslationMethod=None  TranslationStandardOffset=0  TranslationStandardOffsetUnits=m  TranslationStandardAxis=+Z  TranslationCartesianOffset=[0 0 0]  TranslationCartesianOffsetUnits=m  TranslationROffset=0  TranslationROffsetUnits=m  TranslationZOffset=0  TranslationZOffsetUnits=m  TranslationThetaOffset=0  TranslationThetaOffsetUnits=deg  RotationMethod=RotationSequence  RotationAngleUnits=deg  RotationStandardAxis=+X  RotationAngle=180  RotationArbitraryAxis=[0 0 1]  FollAlignAxisA=+X  BaseAlignAxisA=+Y  FollAlignAxisB=+Y  BaseAlignAxisB=+Z  RotationSequenceAxes=BaseAxes  RotationSequence=XYZ  RotationSequenceAngles=[180 0 0]  RotationSequenceAnglesUnits=deg  RotationMatrix=[1 0 0; 0 1 0; 0 0 1]  Quaternion=[1 0 0 0]
  Transform RB2 : sm_lib/Frames and Transforms/Rigid Transform  Commented=through  TranslationMethod=None  TranslationStandardOffset=0  TranslationStandardOffsetUnits=m  TranslationStandardAxis=+Z  TranslationCartesianOffset=[0 0 0]  TranslationCartesianOffsetUnits=m  TranslationROffset=0  TranslationROffsetUnits=m  TranslationZOffset=0  TranslationZOffsetUnits=m  TranslationThetaOffset=0  TranslationThetaOffsetUnits=deg  RotationMethod=RotationSequence  RotationAngleUnits=deg  RotationStandardAxis=+X  RotationAngle=180  RotationArbitraryAxis=[0 0 1]  FollAlignAxisA=+X  BaseAlignAxisA=+Y  FollAlignAxisB=+Y  BaseAlignAxisB=+Z  RotationSequenceAxes=BaseAxes  RotationSequence=XYZ  RotationSequenceAngles=[180 0 90]  RotationSequenceAnglesUnits=deg  RotationMatrix=[1 0 0; 0 1 0; 0 0 1]  Quaternion=[1 0 0 0]
  Transform RF : sm_lib/Frames and Transforms/Rigid Transform  TranslationMethod=None  TranslationStandardOffset=0  TranslationStandardOffsetUnits=m  TranslationStandardAxis=+Z  TranslationCartesianOffset=[0 0 0]  TranslationCartesianOffsetUnits=m  TranslationROffset=0  TranslationROffsetUnits=m  TranslationZOffset=0  TranslationZOffsetUnits=m  TranslationThetaOffset=0  TranslationThetaOffsetUnits=deg  RotationMethod=StandardAxis  RotationAngleUnits=deg  RotationStandardAxis=+Y  RotationAngle=90  RotationArbitraryAxis=[0 0 1]  FollAlignAxisA=+X  BaseAlignAxisA=+Y  FollAlignAxisB=+Y  BaseAlignAxisB=+Z  RotationSequenceAxes=FollowerAxes  RotationSequence=XYX  RotationSequenceAngles=[0 0 0]  RotationSequenceAnglesUnits=deg  RotationMatrix=[1 0 0; 0 1 0; 0 0 1]  Quaternion=[1 0 0 0]
  L : PMIOPort  Side=Left
  R : PMIOPort  Port=2  Side=Right
  connections:
  Transform RB1/LConn1 -- Right Plate/RConn1
  Middle Section/LConn1 -- Left Plate/RConn1
  Left Connector/RConn1 -- Left Plate/LConn1
  Transform LZ/RConn1 -- Left Connector/LConn1
  Right Plate/LConn1 -- Middle Section/RConn1
  Transform LX/LConn1 -- L/RConn1
  Transform RB1/RConn1 -- Transform RB2/LConn1
  Transform RF/LConn1 -- Right Connector/RConn1
  Transform LZ/LConn1 -- Transform LX/RConn1
  Transform RB2/RConn1 -- Right Connector/LConn1
  R/RConn1 -- Transform RF/RConn1

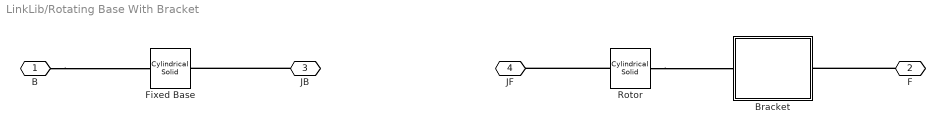
== system LinkLib/Rotating Base With Bracket ==
  Bracket : Subsystem  VariantControl=BracketL  mask{bracketLength=(0.8*baseRadius/2)*1.5, bracketWidth=0.8*baseRadius*0.9, bracketCirclePoints=30, holeRadius=0.8*baseRadius/3, bracketRadius=0.8*baseRadius}
      mask prompts: bracketLength "Bracket length (m)"; bracketWidth "Bracket width (m)"; bracketCirclePoints "Circle resolution"; holeRadius "Hole radius (m)"; bracketRadius "Bracket radius (m)"
      mask Display:
      | image('LinkBracketIcon.png');
      | port_label('lconn',1,'B');
      | port_label('rconn',1,'F');
  Fixed Base : sm_lib/Body Elements/Cylindrical Solid  GraphicAmbientColor=[0.15 0.15 0.15 1.0]  BasedOnType=Density  CenterOfMass=baseCM  CenterOfMassUnits=m  GraphicDiffuseColor=baseColor  CylinderLength=0.025882  CylinderLengthUnits=m  CylinderRadius=baseRadius  CylinderRadiusUnits=m  Density=baseDensity  DensityUnits=kg/m^3  DoExposeReferenceFrame=off  GraphicEmissiveColor=[0.0 0.0 0.0 1.0]  ExportEntireGeometry=off  SerializedFrames=<Frames><Frame><Id>Frame1</Id><Value><Name>F1</Name><Origin><Source>GeometricFeature</Source><FeatureName>bottom surface</FeatureName></Origin><PrimaryAxis><DefinedDirection>+Z</DefinedDirection><Source>ReferenceFrame</Source><SourceDirection>+Z</SourceDirection><FeatureName></FeatureName></PrimaryAxis><SecondaryAxis><DefinedDirection>+X</DefinedDirection><Source>ReferenceFrame</Source><SourceDirection>+X</SourceDirection><FeatureName></FeatureName></SecondaryAxis></Value></Frame><Frame><Id>Frame2</Id><Value><Name>F2</Name><Origin><Source>GeometricFeature</Source><FeatureName>top surface</FeatureName></Origin><PrimaryAxis><DefinedDirection>+Z</DefinedDirection><Source>ReferenceFrame</Source><SourceDirection>+Z</SourceDirection><FeatureName></FeatureName></PrimaryAxis><SecondaryAxis><DefinedDirection>+X</DefinedDirection><Source>ReferenceFrame</Source><SourceDirection>+X</SourceDirection><FeatureName></FeatureName></SecondaryAxis></Value></Frame></Frames>  MarkerShape=Sphere  MarkerSize=10  GraphicType=FromGeometry  InertiaType=Custom  Mass=baseMass  MassUnits=kg  MomentsOfInertia=baseMOI  MomentsOfInertiaUnits=kg*m^2  GraphicOpacity=1.0  ProductsOfInertia=basePOI  ProductsOfInertiaUnits=kg*m^2  GraphicShininess=75  GraphicSpecularColor=[0.5 0.5 0.5 1.0]  GraphicVisPropType=SimpleVisualProperties
  Rotor : sm_lib/Body Elements/Cylindrical Solid  GraphicAmbientColor=[0.15 0.15 0.15 1.0]  BasedOnType=Density  CenterOfMass=rotorCM  CenterOfMassUnits=m  GraphicDiffuseColor=rotorColor  CylinderLength=0.018118  CylinderLengthUnits=m  CylinderRadius=0.8*baseRadius  CylinderRadiusUnits=m  Density=rotorDensity  DensityUnits=kg/m^3  DoExposeReferenceFrame=off  GraphicEmissiveColor=[0.0 0.0 0.0 1.0]  ExportEntireGeometry=off  SerializedFrames=<Frames><Frame><Id>Frame2</Id><Value><Name>F1</Name><Origin><Source>GeometricFeature</Source><FeatureName>bottom surface</FeatureName></Origin><PrimaryAxis><DefinedDirection>+Z</DefinedDirection><Source>ReferenceFrame</Source><SourceDirection>+Z</SourceDirection><FeatureName></FeatureName></PrimaryAxis><SecondaryAxis><DefinedDirection>+X</DefinedDirection><Source>ReferenceFrame</Source><SourceDirection>+X</SourceDirection><FeatureName></FeatureName></SecondaryAxis></Value></Frame><Frame><Id>Frame3</Id><Value><Name>F2</Name><Origin><Source>GeometricFeature</Source><FeatureName>top surface</FeatureName></Origin><PrimaryAxis><DefinedDirection>+Z</DefinedDirection><Source>ReferenceFrame</Source><SourceDirection>+Z</SourceDirection><FeatureName></FeatureName></PrimaryAxis><SecondaryAxis><DefinedDirection>+X</DefinedDirection><Source>ReferenceFrame</Source><SourceDirection>+X</SourceDirection><FeatureName></FeatureName></SecondaryAxis></Value></Frame></Frames>  MarkerShape=Sphere  MarkerSize=10  GraphicType=FromGeometry  InertiaType=Custom  Mass=rotorMass  MassUnits=kg  MomentsOfInertia=rotorMOI  MomentsOfInertiaUnits=kg*m^2  GraphicOpacity=1.0  ProductsOfInertia=rotorPOI  ProductsOfInertiaUnits=kg*m^2  GraphicShininess=75  GraphicSpecularColor=[0.5 0.5 0.5 1.0]  GraphicVisPropType=SimpleVisualProperties
  B : PMIOPort  Side=Left
  F : PMIOPort  Port=2  Side=Right
  JB : PMIOPort  Port=3  Side=Left
  JF : PMIOPort  Port=4  Side=Right
  connections:
  Rotor/LConn1 -- JF/RConn1
  Rotor/RConn1 -- Bracket/LConn1
  F/RConn1 -- Bracket/RConn1
  JB/RConn1 -- Fixed Base/RConn1
  B/RConn1 -- Fixed Base/LConn1
